simulink model "MSC_MATLAB_AGV_ROMB_diploma"  (R2016b)
settings: Solver=VariableStepAuto  StartTime=0.0  StopTime=100  RelTol=1e-3
PreLoadFcn:
  | load('C:\Users\CAD_Admin\AGV\gostask\warehouse1.mat')
  | AGV_Simple_ New
values from neighbouring files (symbols this model uses):
  lns = lns1    [CMDTrackRead.m]    (also in algorithm_test.mat = [1 3 5 7 9 11 13 15 17 19 21 23 ... (242 elements, 121x2)]; warehouseGubkina.mat = [9 3 2 10 4 8 7 3 8 5 7 6 ... (26 elements, 13x2)]; warehouseGubkinaNew.mat = [9 15 17 10 19 11 13 3 3 5 5 8 ... (46 elements, 23x2)])
  pnts = RoundingPnts(pnts)    [Avoidance_Testing.m]    (also in CMDTrackRead.m = pnts1; algorithm_test.mat = [-350 450 0 0 100 100 -340 -260 -100 -100 -350 450 ... (321 ; warehouseGubkina.mat = [4100 4100 4100 3646 3646 3646 3822 3822 4100 4198.5 3822 34; warehouseGubkinaNew.mat = [4100 4100 4100 3646 3646 3646 3822 3822 4100 4198.5 3822 38)
  value0 = [23350 22900 22450 20300 17050 13100 10500 8700 8100 7800 7700 7800 ... (21 elements, 21x1)]    [algorithm_test.mat]
  x0 = 10    [SecondAGV.m]    (also in algorithm_test.mat = [-70 -50 -40 -35 -30 -25 -20 -15 -10 -5 0 5 ... (21 elements)
undefined symbols (not defined in the file): ADAMS_cwd, ADAMS_exec, ADAMS_host, ADAMS_init, ADAMS_inputs, ADAMS_outputs, ADAMS_prefix, ADAMS_static, ADAMS_sysdir
libraries: simulink x7
settings Model: Creator=CAD_Admin  LastModifiedBy=Master

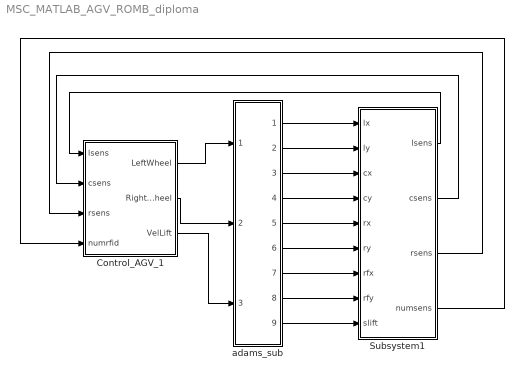
== system MSC_MATLAB_AGV_ROMB_diploma ==
  Control_AGV_1 : Subsystem
  Subsystem1 : Subsystem
  adams_sub : Subsystem
  wires:
  Control_AGV_1/1(LeftWheel) -> adams_sub/1("SEVelLeft ")
  Control_AGV_1/2(RightWheel) -> adams_sub/2(SEVelRight)
  Subsystem1/1(lsens) -> Control_AGV_1/1(lsens)
  Subsystem1/2(csens) -> Control_AGV_1/2(csens)
  Subsystem1/3(rsens) -> Control_AGV_1/3(rsens)
  Subsystem1/4(numsens) -> Control_AGV_1/4(numrfid)
  adams_sub/1("SESensorCLX  ") -> Subsystem1/1(lx)
  adams_sub/2("SESensorCLY  ") -> Subsystem1/2(ly)
  adams_sub/3("SESensorCX   ") -> Subsystem1/3(cx)
  adams_sub/4("SESensorCY   ") -> Subsystem1/4(cy)
  adams_sub/5("SESensorCRX  ") -> Subsystem1/5(rx)
  adams_sub/6("SESensorCRY  ") -> Subsystem1/6(ry)
  adams_sub/7(SESensorRFIDX) -> Subsystem1/7(rfx)
  adams_sub/8(SESensorRFIDY) -> Subsystem1/8(rfy)
  adams_sub/9("SESensorLift ") -> Subsystem1/9(slift)
  Control_AGV_1/3(VelLift) -> adams_sub/3(SEActuator)

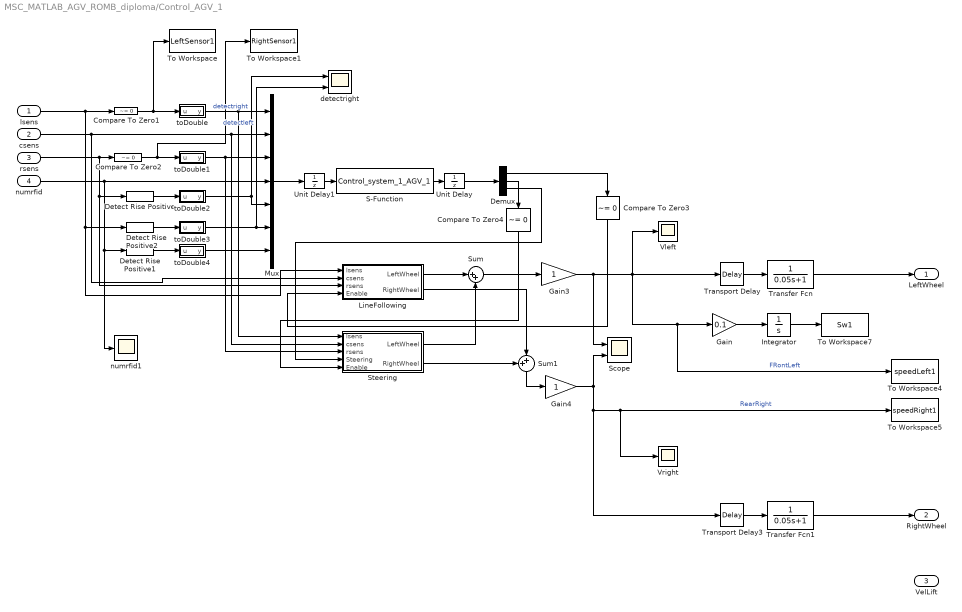
== system MSC_MATLAB_AGV_ROMB_diploma/Control_AGV_1 ==
  lsens : Inport
  csens : Inport  Port=2
  rsens : Inport  Port=3
  numrfid : Inport  Port=4
  Compare To Zero1 : simulink/Logic and Bit Operations/Compare To Zero  relop=~=  OutDataTypeStr=uint8
  Compare To Zero2 : simulink/Logic and Bit Operations/Compare To Zero  relop=~=  OutDataTypeStr=uint8
  Compare To Zero3 : simulink/Logic and Bit Operations/Compare To Zero  relop=~=  OutDataTypeStr=boolean
  Compare To Zero4 : simulink/Logic and Bit Operations/Compare To Zero  relop=~=  OutDataTypeStr=boolean
  Demux : Demux  Outputs=3
  Detect Rise Positive : simulink/Logic and Bit Operations/Detect Rise Positive  vinit=0  OutDataTypeStr=boolean
  Detect Rise Positive1 : simulink/Logic and Bit Operations/Detect Rise Positive  vinit=0  OutDataTypeStr=boolean
  Detect Rise Positive2 : simulink/Logic and Bit Operations/Detect Rise Positive  vinit=0  OutDataTypeStr=boolean
  Gain : Gain  Gain=0.1
  Gain3 : Gain
  Gain4 : Gain
  Integrator : Integrator
  LineFollowing : Subsystem  TreatAsAtomicUnit=on
  Mux : Mux  Inputs=7
  S-Function : S-Function  FunctionName=Control_system_1_AGV_1  Parameters=lns,pnts  SFunctionDeploymentMode=off  EnableBusSupport=off
  Scope : Scope  NumInputPorts=2
  Steering : Subsystem  TreatAsAtomicUnit=on
  Sum : Sum  Inputs=|++
  Sum1 : Sum  Inputs=++|
  To Workspace : ToWorkspace  VariableName=LeftSensor1  SaveFormat=Timeseries  SampleTime=-1
  To Workspace1 : ToWorkspace  VariableName=RightSensor1  SaveFormat=Timeseries  SampleTime=-1
  To Workspace4 : ToWorkspace  VariableName=speedLeft1  SaveFormat=Timeseries  SampleTime=-1
  To Workspace5 : ToWorkspace  VariableName=speedRight1  SaveFormat=Timeseries  SampleTime=-1
  To Workspace7 : ToWorkspace  VariableName=Sw1  SaveFormat=Timeseries  SampleTime=-1
  Transfer Fcn : TransferFcn  Denominator=[0.05 1]
  Transfer Fcn1 : TransferFcn  Denominator=[0.05 1]
  Transport Delay : TransportDelay  DelayTime=0.125
  Transport Delay3 : TransportDelay  DelayTime=0.125
  Unit Delay : UnitDelay  SampleTime=-1
  Unit Delay1 : UnitDelay  SampleTime=-1
  Vleft : Scope
  Vright : Scope
  "detectright " : Scope  NumInputPorts=2
  numrfid1 : Scope
  toDouble : MATLAB Function  TreatAsAtomicUnit=on
  toDouble1 : MATLAB Function  TreatAsAtomicUnit=on
  toDouble2 : MATLAB Function  TreatAsAtomicUnit=on
  toDouble3 : MATLAB Function  TreatAsAtomicUnit=on
  toDouble4 : MATLAB Function  TreatAsAtomicUnit=on
  LeftWheel : Outport
  RightWheel : Outport  Port=2
  VelLift : Outport  Port=3
  wires:
  Gain4/1 -> Transport Delay3/1, Vright/1, To Workspace5/1, Scope/2  "RearRight"
  csens/1 -> LineFollowing/2(csens), Steering/2(csens), Mux/2
  Demux/1 -> Compare To Zero3/1
  Compare To Zero3/1 -> LineFollowing/4(Enable)
  S-Function/1 -> Unit Delay/1
  toDouble/1(y) -> Steering/1(lsens), Mux/1
  toDouble1/1(y) -> Steering/3(rsens), Mux/3
  Compare To Zero4/1 -> Steering/5(Enable)
  Demux/2 -> Compare To Zero4/1
  Steering/1(LeftWheel) -> Sum/2
  Sum/1 -> Gain3/1
  LineFollowing/1(LeftWheel) -> Sum/1
  Steering/2(RightWheel) -> Sum1/1
  Sum1/1 -> Gain4/1
  LineFollowing/2(RightWheel) -> Sum1/2
  Demux/3 -> Steering/4(Steering)
  Unit Delay/1 -> Demux/1
  Detect Rise Positive/1 -> toDouble2/1(u)
  toDouble2/1(y) -> Mux/5, "detectright "/1  "detectright"
  Detect Rise Positive1/1 -> toDouble4/1(u)
  toDouble4/1(y) -> Mux/7
  toDouble3/1(y) -> "detectright "/2, Mux/6  "detectleft"
  Detect Rise Positive2/1 -> toDouble3/1(u)
  Mux/1 -> Unit Delay1/1
  Unit Delay1/1 -> S-Function/1
  Compare To Zero1/1 -> To Workspace/1, toDouble/1(u)
  Compare To Zero2/1 -> To Workspace1/1, toDouble1/1(u)
  lsens/1 -> LineFollowing/1(lsens), Detect Rise Positive2/1, Compare To Zero1/1
  rsens/1 -> LineFollowing/3(rsens), Detect Rise Positive/1, Compare To Zero2/1
  Gain3/1 -> Scope/1, Transport Delay/1, Vleft/1, Gain/1, To Workspace4/1  "FRontLeft"
  Transport Delay/1 -> Transfer Fcn/1
  Transport Delay3/1 -> Transfer Fcn1/1
  Transfer Fcn1/1 -> RightWheel/1
  numrfid/1 -> Detect Rise Positive1/1, numrfid1/1, Mux/4
  Gain/1 -> Integrator/1
  Integrator/1 -> To Workspace7/1
  Transfer Fcn/1 -> LeftWheel/1

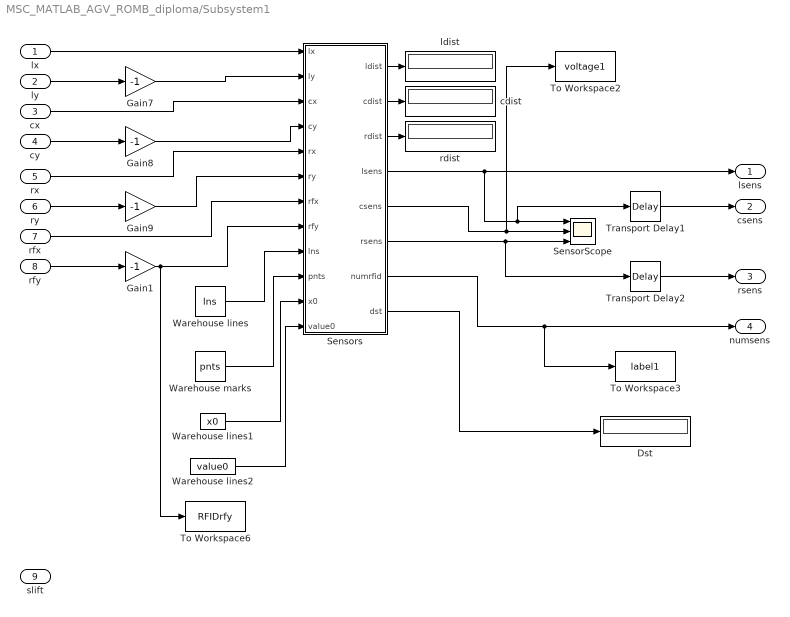
== system MSC_MATLAB_AGV_ROMB_diploma/Subsystem1 ==
  lx : Inport
  ly : Inport  Port=2
  cx : Inport  Port=3
  cy : Inport  Port=4
  rx : Inport  Port=5
  ry : Inport  Port=6
  rfx : Inport  Port=7
  rfy : Inport  Port=8
  slift : Inport  Port=9
  Dst : Display
  Gain{1,7..9} (4 alike) : Gain  Gain=-1
  SensorScope : Scope  NumInputPorts=3
  Sensors : MATLAB Function  TreatAsAtomicUnit=on
  To Workspace2 : ToWorkspace  VariableName=voltage1  SaveFormat=Timeseries  SampleTime=-1
  To Workspace3 : ToWorkspace  VariableName=label1  SaveFormat=Timeseries  SampleTime=-1
  To Workspace6 : ToWorkspace  VariableName=RFIDrfy  SaveFormat=Timeseries  SampleTime=-1
  Transport Delay1 : TransportDelay  DelayTime=0.3
  Transport Delay2 : TransportDelay  DelayTime=0.3
  Warehouse lines : Constant  Value=lns  VectorParams1D=off
  Warehouse lines1 : Constant  Value=x0  VectorParams1D=off
  Warehouse lines2 : Constant  Value=value0  VectorParams1D=off
  Warehouse marks : Constant  Value=pnts  VectorParams1D=off
  cdist : Display
  ldist : Display
  rdist : Display
  lsens : Outport
  csens : Outport  Port=2
  rsens : Outport  Port=3
  numsens : Outport  Port=4
  wires:
  cy/1 -> Gain8/1
  cx/1 -> Sensors/3(cx)
  lx/1 -> Sensors/1(lx)
  rx/1 -> Sensors/5(rx)
  Warehouse marks/1 -> Sensors/10(pnts)
  Sensors/1(ldist) -> ldist/1
  Sensors/2(cdist) -> cdist/1
  Sensors/3(rdist) -> rdist/1
  ly/1 -> Gain7/1
  Gain7/1 -> Sensors/2(ly)
  Gain8/1 -> Sensors/4(cy)
  Gain9/1 -> Sensors/6(ry)
  Sensors/5(csens) -> To Workspace2/1, SensorScope/2
  Sensors/8(dst) -> Dst/1
  Warehouse lines/1 -> Sensors/9(lns)
  ry/1 -> Gain9/1
  rfx/1 -> Sensors/7(rfx)
  Gain1/1 -> Sensors/8(rfy), To Workspace6/1
  rfy/1 -> Gain1/1
  Sensors/4(lsens) -> SensorScope/1, Transport Delay1/1, lsens/1
  Sensors/6(rsens) -> SensorScope/3, Transport Delay2/1
  Warehouse lines1/1 -> Sensors/11(x0)
  Warehouse lines2/1 -> Sensors/12(value0)
  Sensors/7(numrfid) -> numsens/1, To Workspace3/1
  Transport Delay1/1 -> csens/1
  Transport Delay2/1 -> rsens/1

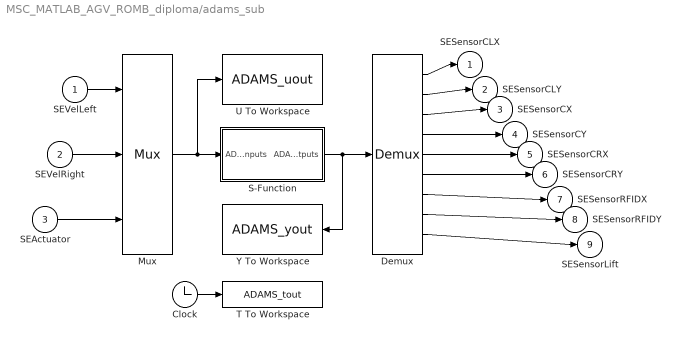
== system MSC_MATLAB_AGV_ROMB_diploma/adams_sub ==
  "SEVelLeft " : Inport
  SEVelRight : Inport  Port=2
  SEActuator : Inport  Port=3
  Clock : Clock
  Demux : Demux  Outputs=9
  Mux : Mux  Inputs=3
  S-Function : Subsystem  LoadFcn=|  InitFcn=clear mex  mask(Adams Plant){exevie=ADAMS_sysdir, nam_in=ADAMS_inputs, namout=ADAMS_outputs, nampre=ADAMS_prefix, outfil=ADAMS_prefix, exesol=ADAMS_exec, stat=ADAMS_static, inicmd=[ADAMS_init], exetyp=C++, comtyp=PIPE(DDE), workdir=ADAMS_cwd, ada_host=ADAMS_host, modani=batch, modsim=discrete, dft=no, simulink_lead_cosim=yes, pin_interp_order=0, pout_extrap_order=0, pin_extrap_order=0, pout_interp_order=0, dt_out=0.005, o_rate=1, more=off}
      | %check based on dialog box setting for when setting by popup menu                                             
      | if exist('ADAMS_solver_type')                                                                                 
      |   if strcmp(ADAMS_solver_type,'C++')                                                                          
      |     set_param(gcb,'exetyp','C++');                                                                            
      |   else                                                                                                        
      |     set_param(gcb,'exetyp','Fortran');                                                                        
      |   end                                                                                                         
      | else                                                                                                          
      |   set_param(gcb,'exetyp','C++');                                                                              
      | end                                                                                                           
      | %set the mode if using acar_solver                                                                            
      | %REQUIRED HERE BECAUSE BELOW CAUSES MDLTERMINATE TO BE CALLED 2 TIMES IN MIDDLE OF SIMULATION WHEN SET IN MASK
      |                                                                                                               
      | %enable the direct feedthrough, sim mode, anim mode parameters by default                                     
      |                                                                                                               
      | if exist('set_some_params_states')                                                                            
      |                                                                                                               
      |   set_some_params_states({'dft','modsim','modani'},{'on','on','on'},'MaskEnables',gcb)                        
      |   %turn on direct feedthrough option                                                                          
      |   set_some_params_states({'dft'},{'on'},'MaskVisibilities',gcb)                                               
      |                                                                                                               
      |  end                                                                                                          
      |                                                                                                               
      |                                                                                                               
      | if exist('ADAMS_exec')                                                                                        
      |   if and(strcmp(get_param(gcb,'exesol'),'ADAMS_exec'),strcmp(ADAMS_exec,'acar_solver'))                       
      |     %set the sim mode to discrete -- only supported mode                                                      
      |     set_param(gcb,'modsim','discrete')                                                                        
      |      %turn off direct feedthrough option                                                                      
      |      set_some_params_states({'dft'},{'off'},'MaskVisibilities',gcb)                                           
      |     %set the animation mode to batch -- only supported mode                                                   
      |     set_param(gcb,'modani','batch')                                                                           
      |     %disable the direct feedthrough, sim mode, anim mode parameters                                           
      |     set_some_params_states({'modsim','modani'},{'off','off'},'MaskEnables',gcb)                               
      |   end                                                                                                         
      | end
      mask prompts: exevie "Adams install directory"; nam_in "Adams/View input names"; namout "Adams/View output names"; nampre "Adams model file prefix"; outfil "Output files prefix (opt.: if blank - no output)"; exesol "User executable (opt.: if blank - use standard)"; stat "Initial static simulation flag"; inicmd "Initialization commands"; exetyp "Adams/Solver type"; comtyp "Interprocess option"; workdir "Adams working directory"; ada_host "Adams host"; modani "Animation mode"; modsim "Simulation mode"; dft "Direct feedthrough"; simulink_lead_cosim "Discrete Computational Order - Simulink Leads Adams"; pin_interp_order "Plant input interpolation order"; pout_extrap_order "Plant output extrapolation order"; pin_extrap_order "Plant input extrapolation order"; pout_interp_order "Plant output interpolation order"; dt_out "Communication interval"; o_rate "Number of communications per output step"; more "More parameters"
      mask help: Simulate any Adams plant model either in Adams/Solver form (.adm file) or in Adams/View form (.cmd file)
      settings: OpenFcn=|
      | open_system(gcb,'mask')
      | if not(exist('set_some_params_states'))
      | 
      | warning('The script "set_some_params_states.m" cannot be found in the MATLAB PATH.  Cannot update the ADAMS Plant S-Function parameters.')
      | 
      | warning('Recommended action(optional):  run the Adams/Controls .m file first to help choose the correct settings in the Adams S-Function block.')
      | 
      | end
      mask Help:
      | <html>
      | This S-Function represents the non-linear Adams Plant with the inputs sent to the Adams model <br>
      |  and the outputs generated by the Adams model.  See the Adams/Controls documentation for more <br>
      | information.  This plant uses the following variables:<br>
      | <br>
      | <b>ADAMS_sysdir  :</b> Adams installation directory<br>
      | <b>ADAMS_inputs  :</b> Input variables View names vector<br>
      | <b>ADAMS_outputs :</b> Outputs variables View names vector<br>
      | <b>ADAMS_prefix  : </b>ADAMS model files prefix (.adm, .cmd); also doubles as output files prefix<br>
      | <b>ADAMS_exec :</b> Adams/Solver user library or keyword (e.g., acar_solver)<br>
      | <b>ADAMS_static :</b> yes|no - initial static before Co-simulation(discrete)/Function Evaluation(continuous)<br>
      | <b>ADAMS_init :</b>Initialization commands (i.e., Adams/View or Solver commands, depending on setting for Animation mode)<br>
      | <b>ADAMS_cwd : </b> Current working directory (for TCP/IP)<br>
      | <b>ADAMS_host : </b>Name of Adams server host (for TCP/IP)<br>
      | <b>ADAMS_mode :</b> Linear or non-linear (i.e., co-sim, function eval)<br>
      | <b>ADAMS_solver_type :</b>Fortran or C++ (used to set popup menu when first loaded) <br>
      | 
      | 
      | <br>
      | The following settings can be chosen:<br>
      | <br>
      | <b>Adams/Solver type:</b>  Fortran or C++ (will also set ADAMS_solver_type)<br>
      | <b>Interprocess option:</b> Pipe(DDE) or TCP/IP; TCP/IP can allow different machines run Adams and MATLAB<br>
      | <b>Animation mode:</b> batch (Solver, uses .adm) or interactive (View, uses .cmd)<br>
      | <b>Simulation mode:</b> discrete (Co-simulation) or continuous (Function Evaluation)<br>
      | <b>Discrete Computational Order - Simulink Lead Adams:</b> for discrete mode, chooses if Simulink leads the integration (yes) or lags (no);<br> if set to "no", can remove algebraic loop<br>
      | <b>Plant input interpolation order:</b> 0 = zero-order hold; 1 = linear (discrete mode only, where Simulink leads)<br>
      | <b>Plant output extrapolation order:</b> 0 = zero-order hold;1 = linear(discrete mode only, where Simulink leads)<br>
      | <b>Plant input extrapolation order:</b> 0 = zero-order hold; 1 = linear (discrete mode only, where Adams leads)<br>
      | <b>Plant output interpolation order:</b> 0 = zero-order hold;1 = linear(discrete mode only, where Adams leads)<br>
      | <b>Direct feedthrough:</b> yes|no - yes = Input directly effect output(continuous mode-only)<br>
      | <b>Communication interval:</b> Time step at which Co-simulation exchange information (e.g.,0.005); also controls <br>output for continuous mode (Function Evaluation)<br>
      | <b>Number of communications per output step: </b>Sets Adams output rate (.res, .req, .gra) integer value (default: 1)<br>
      | </html>
      mask Callback exesol:
      | if exist('set_some_params_states')
      | %enable the direct feedthrough, sim mode, anim mode parameters
      | set_some_params_states({'dft','modsim','modani'},{'on','on','on'},'MaskEnables',gcb)
      | %turn on direct feedthrough option
      | set_some_params_states({'dft'},{'on'},'MaskVisibilities',gcb)
      | end
      | 
      | if exist('ADAMS_exec')
      |   if and(strcmp(get_param(gcb,'exesol'),'ADAMS_exec'),strcmp(ADAMS_exec,'acar_solver'))
      |     %set the sim mode to discrete -- only supported mode
      |     %REMOVED:  BELOW CAUSES MDLTERMINATE TO BE CALLED 2 TIMES IN MIDDLE OF SIMULATION
      |     %Now in LoadFcn callback
      |     %set_param(gcb,'modsim','discrete')
      |      %turn off direct feedthrough option
      |     set_some_params_states({'dft'},{'off'},'MaskVisibilities',gcb)
      |     %set the animation mode to batch -- only supported mode
      |     %REMOVED:  BELOW CAUSES MDLTERMINATE TO BE CALLED 2 TIMES IN MIDDLE OF SIMULATION
      |     %Now in LoadFcn callback
      |     %set_param(gcb,'modani','batch')
      |     %disable the direct feedthrough, sim mode, anim mode parameters
      |     set_some_params_states({'modsim','modani'},{'off','off'},'MaskEnables',gcb)
      |   end
      | end
      mask TypeOptions exetyp: Fortran | C++
      mask Callback exetyp:
      | if strcmp(get_param(gcb,'exetyp'),'C++')
      |     ADAMS_solver_type='C++';
      | else
      |     ADAMS_solver_type='Fortran';
      | end
      mask TypeOptions comtyp: PIPE(DDE) | TCP/IP
      mask Callback comtyp:
      | if exist('set_some_params_states')
      | if strcmp(get_param(gcb,'comtyp'),'PIPE(DDE)')
      |     %turn off cwd, host options
      |     set_some_params_states({'ada_host','workdir'},{'off','off'},'MaskVisibilities',gcb)
      | else%if strcmp(get_param(gcb,'modsim'),'TCP/IP')
      |     %turn on cwd, host options
      |     set_some_params_states({'ada_host','workdir'},{'on','on'},'MaskVisibilities',gcb)
      | end
      | end
      mask TypeOptions modani: batch | interactive
      mask TypeOptions modsim: discrete | continuous
      mask Callback modsim:
      | if exist('set_some_params_states')
      | if strcmp(get_param(gcb,'modsim'),'discrete')
      |      %turn off direct feedthrough option
      |     set_some_params_states({'dft'},{'off'},'MaskVisibilities',gcb)
      |     %turn on discrete co-sim type if want to see more
      |     if strcmp(get_param(gcb,'more'),'on')
      |         set_some_params_states({'simulink_lead_cosim'},{'on'},'MaskVisibilities',gcb)
      |     end
      |     if strcmp(get_param(gcb,'simulink_lead_cosim'),'yes')
      |         %turn on interpolation/extrapolation options
      |         set_some_params_states({'pin_interp_order','pout_extrap_order',},{'on','on'},'MaskVisibilities',gcb)
      |     else
      |         set_some_params_states({'pin_extrap_order','pout_interp_order'},{'on','on'},'MaskVisibilities',gcb)
      |     end
      | else%if strcmp(get_param(gcb,'modsim'),'continuous')
      |      %turn off direct feedthrough option
      |     set_some_params_states({'dft'},{'on'},'MaskVisibilities',gcb)
      |     %turn off interpolation/extrapolation options
      |     set_some_params_states({'pin_interp_order','pout_extrap_order','pin_extrap_order','pout_interp_order','simulink_lead_cosim'},{'off','off','off','off','off'},'MaskVisibilities',gcb)
      | end
      | end
      mask TypeOptions dft: no | yes
      mask TypeOptions simulink_lead_cosim: yes | no
      mask Callback simulink_lead_cosim:
      | if exist('set_some_params_states')
      | if (strcmp(get_param(gcb,'simulink_lead_cosim'),'yes') && strcmp(get_param(gcb,'modsim'),'discrete'))
      |      %turn off unused interpolate/extrapolate options
      |     set_some_params_states({'pin_extrap_order','pout_interp_order'},{'off','off'},'MaskVisibilities',gcb)
      |     %turn on used interpolate/extrapolate options
      |     set_some_params_states({'pin_interp_order','pout_extrap_order'},{'on','on'},'MaskVisibilities',gcb)
      | elseif (strcmp(get_param(gcb,'simulink_lead_cosim'),'no') && strcmp(get_param(gcb,'modsim'),'discrete'))
      |     %turn on used interpolate/extrapolate options
      |     set_some_params_states({'pin_extrap_order','pout_interp_order'},{'on','on'},'MaskVisibilities',gcb)
      |      %turn off unused interpolate/extrapolate options
      |     set_some_params_states({'pin_interp_order','pout_extrap_order'},{'off','off'},'MaskVisibilities',gcb)
      | end
      | end
      mask TypeOptions pin_interp_order: 0 | 1
      mask TypeOptions pout_extrap_order: 0 | 1
      mask TypeOptions pin_extrap_order: 0 | 1
      mask TypeOptions pout_interp_order: 0 | 1
      mask Callback more:
      | if exist('set_some_params_states')
      | if (strcmp(get_param(gcb,'more'),'on'))
      |      %turn on infrequently used options
      |     set_some_params_states({'exevie','nam_in','namout','exesol','stat','inicmd'},{'on','on','on','on','on','on'},'MaskVisibilities',gcb)
      |     if strcmp(get_param(gcb,'modsim'),'discrete')
      |         set_some_params_states({'simulink_lead_cosim'},{'on'},'MaskVisibilities',gcb)
      |     end
      | elseif (strcmp(get_param(gcb,'more'),'off'))
      |     %turn off infrequently used options
      |     set_some_params_states({'exevie','nam_in','namout','exesol','stat','inicmd'},{'off','off','off','off','off','off'},'MaskVisibilities',gcb)
      |     if strcmp(get_param(gcb,'modsim'),'discrete')
      |         set_some_params_states({'simulink_lead_cosim'},{'off'},'MaskVisibilities',gcb)
      |     end
      | end
      | end
      mask Display: disp( 'MSC Software' )
  T To Workspace : ToWorkspace  VariableName=ADAMS_tout
      settings: MaxDataPoints=100000
  U To Workspace : ToWorkspace  VariableName=ADAMS_uout
      settings: MaxDataPoints=100000
  Y To Workspace : ToWorkspace  VariableName=ADAMS_yout
      settings: MaxDataPoints=100000
  "SESensorCLX  " : Outport
  "SESensorCLY  " : Outport  Port=2
  "SESensorCX   " : Outport  Port=3
  "SESensorCY   " : Outport  Port=4
  "SESensorCRX  " : Outport  Port=5
  "SESensorCRY  " : Outport  Port=6
  SESensorRFIDX : Outport  Port=7
  SESensorRFIDY : Outport  Port=8
  "SESensorLift " : Outport  Port=9
  wires:
  Clock/1 -> T To Workspace/1
  Mux/1 -> S-Function/1(ADAMS inputs), U To Workspace/1
  S-Function/1(ADAMS outputs) -> Demux/1, Y To Workspace/1
  Demux/1 -> "SESensorCLX  "/1
  Demux/2 -> "SESensorCLY  "/1
  Demux/3 -> "SESensorCX   "/1
  Demux/4 -> "SESensorCY   "/1
  Demux/5 -> "SESensorCRX  "/1
  Demux/6 -> "SESensorCRY  "/1
  Demux/7 -> SESensorRFIDX/1
  Demux/8 -> SESensorRFIDY/1
  Demux/9 -> "SESensorLift "/1
  "SEVelLeft "/1 -> Mux/1
  SEVelRight/1 -> Mux/2
  SEActuator/1 -> Mux/3

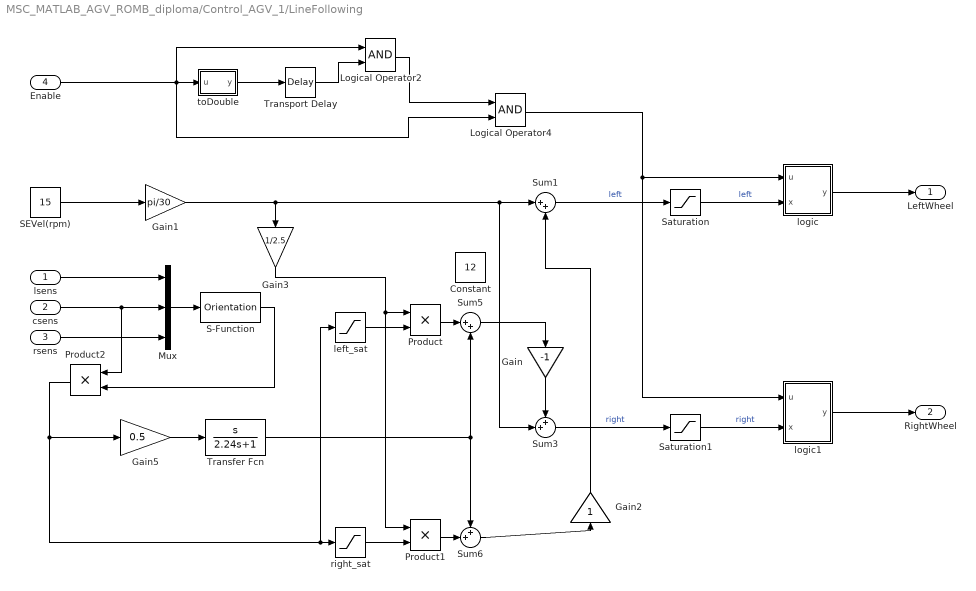
== system MSC_MATLAB_AGV_ROMB_diploma/Control_AGV_1/LineFollowing ==
  lsens : Inport
  csens : Inport  Port=2
  rsens : Inport  Port=3
  Enable : Inport  Port=4
  Constant : Constant  Value=12
  Gain : Gain  Gain=-1
  Gain1 : Gain  Gain=pi/30
  Gain2 : Gain
  Gain3 : Gain  Gain=1/2.5
  Gain5 : Gain  Gain=0.5
  Logical Operator2 : Logic  AllPortsSameDT=off  OutDataTypeStr=boolean
  Logical Operator4 : Logic  AllPortsSameDT=off  OutDataTypeStr=boolean
  Mux : Mux  Inputs=3
  Product : Product
  Product1 : Product
  Product2 : Product
  S-Function : S-Function  FunctionName=Orientation  SFunctionDeploymentMode=off  EnableBusSupport=off
  SEVel(rpm) : Constant  Value=15
  Saturation : Saturate  UpperLimit=inf  LowerLimit=0
  Saturation1 : Saturate  UpperLimit=inf  LowerLimit=0
  Sum1 : Sum  Inputs=|++
  Sum3 : Sum  Inputs=++|
  Sum5 : Sum  Inputs=|++
  Sum6 : Sum  Inputs=++|
  Transfer Fcn : TransferFcn  Numerator=[1 0]  Denominator=[2.24 1]
  Transport Delay : TransportDelay  DelayTime=0.05
  left_sat : Saturate  UpperLimit=0  LowerLimit=-10
  logic : MATLAB Function  TreatAsAtomicUnit=on
  logic1 : MATLAB Function  TreatAsAtomicUnit=on
  right_sat : Saturate  UpperLimit=10  LowerLimit=0
  toDouble : MATLAB Function  TreatAsAtomicUnit=on
  LeftWheel : Outport
  RightWheel : Outport  Port=2
  wires:
  SEVel(rpm)/1 -> Gain1/1
  Gain1/1 -> Sum3/2, Sum1/1, Gain3/1
  lsens/1 -> Mux/1
  rsens/1 -> Mux/3
  Sum6/1 -> Gain2/1
  S-Function/1 -> Product2/2
  csens/1 -> Product2/1, Mux/2
  Product2/1 -> Gain5/1, left_sat/1, right_sat/1
  Saturation/1 -> logic/2(x)  "left"
  logic/1(y) -> LeftWheel/1
  Saturation1/1 -> logic1/2(x)  "right"
  logic1/1(y) -> RightWheel/1
  Logical Operator2/1 -> Logical Operator4/1
  Enable/1 -> Logical Operator2/1, toDouble/1(u), Logical Operator4/2
  toDouble/1(y) -> Transport Delay/1
  Transport Delay/1 -> Logical Operator2/2
  Logical Operator4/1 -> logic1/1(u), logic/1(u)
  Mux/1 -> S-Function/1
  Gain/1 -> Sum3/1
  Gain2/1 -> Sum1/2
  Sum5/1 -> Gain/1
  Gain3/1 -> Product1/1, Product/1
  right_sat/1 -> Product1/2
  left_sat/1 -> Product/2
  Gain5/1 -> Transfer Fcn/1
  Transfer Fcn/1 -> Sum6/1, Sum5/2
  Product/1 -> Sum5/1
  Product1/1 -> Sum6/2
  Sum3/1 -> Saturation1/1  "right"
  Sum1/1 -> Saturation/1  "left"

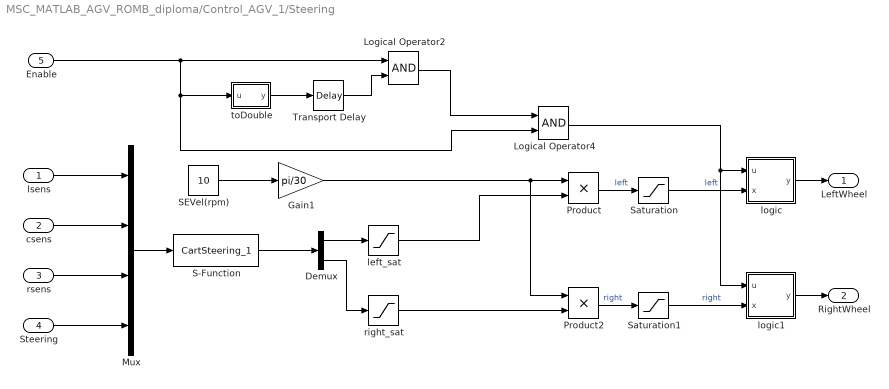
== system MSC_MATLAB_AGV_ROMB_diploma/Control_AGV_1/Steering ==
  lsens : Inport
  csens : Inport  Port=2
  rsens : Inport  Port=3
  Steering : Inport  Port=4
  Enable : Inport  Port=5
  Demux : Demux  Outputs=2
  Gain1 : Gain  Gain=pi/30
  Logical Operator2 : Logic  AllPortsSameDT=off  OutDataTypeStr=boolean
  Logical Operator4 : Logic  AllPortsSameDT=off  OutDataTypeStr=boolean
  Mux : Mux
  Product : Product
  Product2 : Product
  S-Function : S-Function  FunctionName=CartSteering_1  Parameters=lns,pnts  SFunctionDeploymentMode=off  EnableBusSupport=off
  SEVel(rpm) : Constant  Value=10
  Saturation : Saturate  UpperLimit=inf  LowerLimit=-inf
  Saturation1 : Saturate  UpperLimit=inf  LowerLimit=-inf
  Transport Delay : TransportDelay  DelayTime=0.2
  left_sat : Saturate  UpperLimit=2  LowerLimit=-2
  logic : MATLAB Function  TreatAsAtomicUnit=on
  logic1 : MATLAB Function  TreatAsAtomicUnit=on
  right_sat : Saturate  UpperLimit=2  LowerLimit=-2
  toDouble : MATLAB Function  TreatAsAtomicUnit=on
  LeftWheel : Outport
  RightWheel : Outport  Port=2
  wires:
  rsens/1 -> Mux/3
  csens/1 -> Mux/2
  lsens/1 -> Mux/1
  Steering/1 -> Mux/4
  Product/1 -> Saturation/1  "left"
  SEVel(rpm)/1 -> Gain1/1
  Product2/1 -> Saturation1/1  "right"
  Gain1/1 -> Product2/1, Product/1
  Saturation/1 -> logic/2(x)  "left"
  Saturation1/1 -> logic1/2(x)  "right"
  Demux/1 -> left_sat/1
  Demux/2 -> right_sat/1
  Mux/1 -> S-Function/1
  S-Function/1 -> Demux/1
  left_sat/1 -> Product/2
  right_sat/1 -> Product2/2
  logic/1(y) -> LeftWheel/1
  logic1/1(y) -> RightWheel/1
  Logical Operator4/1 -> logic1/1(u), logic/1(u)
  Logical Operator2/1 -> Logical Operator4/1
  Enable/1 -> toDouble/1(u), Logical Operator4/2, Logical Operator2/1
  toDouble/1(y) -> Transport Delay/1
  Transport Delay/1 -> Logical Operator2/2

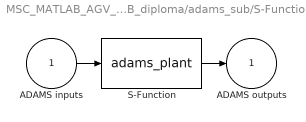
== system MSC_MATLAB_AGV_ROMB_diploma/adams_sub/S-Function ==
  ADAMS inputs : Inport
  S-Function : S-Function  StopFcn=clear mex  FunctionName=adams_plant  Parameters=exevie,exesol,stat,outfil,nampre,o_rate,nam_in,namout,dft,modsim,modani,dt_out,inicmd,exetyp,comtyp,ada_host, workdir,pin_interp_order,pout_extrap_order,pin_extrap_order,pout_interp_order,simulink_lead_cosim  SFunctionDeploymentMode=off  EnableBusSupport=off
  ADAMS outputs : Outport  InitialOutput=0
  wires:
  S-Function/1 -> ADAMS outputs/1
  ADAMS inputs/1 -> S-Function/1

== matlab function MSC_MATLAB_AGV_ROMB_diploma/Control_AGV_1/LineFollowing/logic ==
  data: u input; y output; x input
function y = fcn(u, x)
if (u == true)
    y = x;
else
    y = 0;
end;

== matlab function MSC_MATLAB_AGV_ROMB_diploma/Control_AGV_1/LineFollowing/logic1 ==
  data: u input; y output; x input
function y = fcn(u, x)
if (u == true)
    y = x;
else
    y = 0;
end;

== matlab function MSC_MATLAB_AGV_ROMB_diploma/Control_AGV_1/LineFollowing/toDouble ==
  data: u input; y output
function y = fcn(u)

y = double(u);

== matlab function MSC_MATLAB_AGV_ROMB_diploma/Control_AGV_1/Steering/logic ==
  data: u input; y output; x input
function y = fcn(u, x)
if (u == true)
    y = x;
else
    y = 0;
end;

== matlab function MSC_MATLAB_AGV_ROMB_diploma/Control_AGV_1/Steering/logic1 ==
  data: u input; y output; x input
function y = fcn(u, x)
if (u == true)
    y = x;
else
    y = 0;
end;

== matlab function MSC_MATLAB_AGV_ROMB_diploma/Control_AGV_1/Steering/toDouble ==
  data: u input; y output
function y = fcn(u)

y = double(u);

== matlab function MSC_MATLAB_AGV_ROMB_diploma/Control_AGV_1/toDouble ==
  data: u input; y output
function y = fcn(u)

y = double(u);

== matlab function MSC_MATLAB_AGV_ROMB_diploma/Control_AGV_1/toDouble1 ==
  data: u input; y output
function y = fcn(u)

y = double(u);

== matlab function MSC_MATLAB_AGV_ROMB_diploma/Control_AGV_1/toDouble2 ==
  data: u input; y output
function y = fcn(u)

y = double(u);

== matlab function MSC_MATLAB_AGV_ROMB_diploma/Control_AGV_1/toDouble3 ==
  data: u input; y output
function y = fcn(u)

y = double(u);

== matlab function MSC_MATLAB_AGV_ROMB_diploma/Control_AGV_1/toDouble4 ==
  data: u input; y output
function y = fcn(u)

y = double(u);

== matlab function MSC_MATLAB_AGV_ROMB_diploma/Subsystem1/Sensors ==
  data: lx input; ldist output; ly input; cx input; cy input; rx input; ry input; rfx input; rfy input; lns input; pnts input; cdist output; rdist output; lsens output; csens output; rsens output; numrfid output; dst output; x0 input; value0 input
function [ldist, cdist, rdist, lsens, csens, rsens, numrfid, dst] = fcn(lx, ly, cx, cy, rx, ry, rfx, rfy, lns, pnts, x0, value0)

p00 = [4100 0 -2196];          % Center of coordinates (Matlab)

lpoint = [lx 0 ly] + p00;      % Coordinate of left sensor (Adams to Matlab)  
cpoint = [cx 0 cy] + p00;      % Coordinate of center sensor (Adams to Matlab)  
rpoint = [rx 0 ry] + p00;      % Coordinate of right sensor (Adams to Matlab)  
rfpoint = [rfx 0 rfy] + p00;   % Coordinate of RFID reader (Adams to Matlab) rfy - 50

ldist = min(DistanceLinePoint(pnts,lns,lpoint));
cdist = min(DistanceLinePoint(pnts,lns,cpoint));
rdist = min(DistanceLinePoint(pnts,lns,rpoint));

if (ldist >= 3) 
    lsens = 0;
else
    lsens = 1;
end;

if (rdist >= 3) 
    rsens = 0;
else
    rsens = 1;
end;

%if (cdist >= 5.81) 
  %  csens = 5.81;
%else
  %  csens=cdist;
%end;
% csens = 2.8801 - 1.266 * exp( - ( ( cdist * 10 ) ^ 2 / 612.0676 ) ) - 1.5;
csens = ((interp1(x0,value0, cdist * 10,'linear',23350) - min(value0)) / 32767 ) * 4.096 + 0.05;

% if csens < 0 
%     Psy = 1;
% end

%numrfid=0;
[dst,numrfid] = min(DistancePointPoint(pnts,rfpoint));
if (dst > 3) % before 15ss % after 45
    numrfid = 0;
end;
